simulink model "example_CondensingBoiler"  (R2016b)
settings: Solver=ode45  StartTime=0.0  StopTime=1*24*3600  MaxStep=600  RelTol=1e-4  AbsTol=1e-5  EnableMultiTasking=on
libraries: carnot x6, simulink x2
settings Model: Creator=drhf  LastModifiedBy=drhf
settings DataIOCC: LimitDataPoints=on  SaveFormat=Array
settings OptimizationCC: DefaultParameterBehavior=Inlined  ExpressionDepthLimit=2147483647  LifeSpan=inf
settings DebuggingCC: SolverPrmCheckMsg=warning  UniqueDataStoreMsg=error  StateNameClashWarn=warning  SFUnexpectedBacktrackingDiag=warning  SFNoUnconditionalDefaultTransitionDiag=warning  SFExecutionAtInitializationDiag=none
settings HardwareCC: ProdBitPerPointer=32  ProdBitPerSizeT=32  ProdBitPerPtrDiffT=32  ProdLargestAtomicFloat=None  ProdIntDivRoundTo=Undefined  ProdEndianess=Unspecified  ProdWordSize=32  ProdHWDeviceType=32-bit Generic
settings ModelReferenceCC: PropagateSignalLabelsOutOfModel=off
settings GRTTargetCC: TargetLangStandard=C89/C90 (ANSI)  GeneratePreprocessorConditionals=Disable all  CombineOutputUpdateFcns=off  GRTInterface=on
settings ConfigComp: CovMetricSettings=dw  CovHtmlReporting=on  CovSaveCumulativeToWorkspaceVar=on  CovSaveSingleToWorkspaceVar=on  CovExternalEMLEnable=off

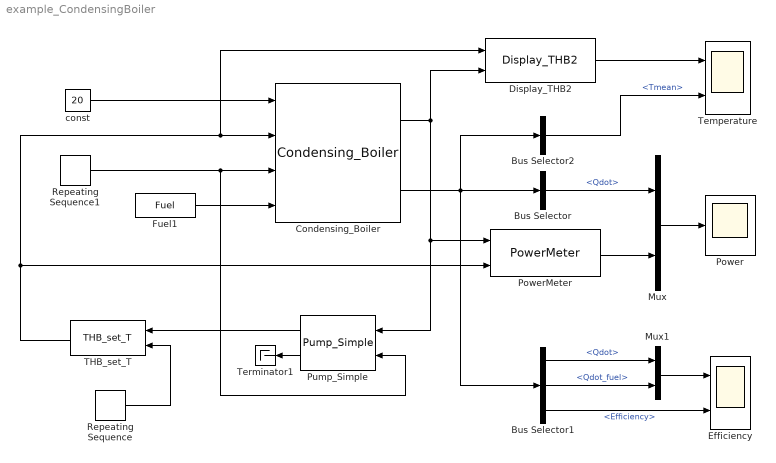
== system example_CondensingBoiler ==
  Bus Selector : BusSelector  OutputSignals=Qdot
  Bus Selector1 : BusSelector  OutputSignals=Qdot,eco.Qdot_fuel,eco.Efficiency
  Bus Selector2 : BusSelector  OutputSignals=Tmean
  Condensing_Boiler : carnot/Source/Boiler/Condensing_Boiler  Pgas=20e3  U=3  vol=0.02  electricPower=[20 120]  relativeQdot=[0.25 1]  whichTforEfficiency=mean of inlet and outlet temperature  temperatures="[40  70]"  efficiency=[1.05 0.95; 1.0 0.9]  lin=10  qua=100  Tini=20  nodes=1
  Display_THB2 : carnot/Outputs/Display_THB2  t=on  m=off  p=off  id=off  mix=off  d=off
  Efficiency : Scope  NumInputPorts=2
  Fuel1 : carnot/Source/Energy/Fuel  ft=1  t=20  ls=1  p=1e5  h_values=[5.14e7 5.69e7]  tc=45  price=1  mass=[0.33 0.67 0 0 0 0]
  Mux : Mux  Inputs=2
  Mux1 : Mux  Inputs=2
  Power : Scope
  PowerMeter : carnot/Control/PowerMeter
  Pump_Simple : carnot/Hydraulics/Pump_Simple  mdotmax=1600/3600  dia=0.0157  power=30  fluid_id=Water  mix=0  p0=3e5
  Repeating Sequence : simulink/Sources/Repeating Sequence  rep_seq_t=[0 12 24]*3600  rep_seq_y=[30 70 30]
  Repeating Sequence1 : simulink/Sources/Repeating Sequence  rep_seq_t=[0 6 12]*3600  rep_seq_y=[1 1 1] %[0.25 1 0.25]
  THB_set_T : carnot/Source/Simple/THB_set_T
  Temperature : Scope  NumInputPorts=2
  Terminator1 : Terminator
  const : Constant  Value=20
  wires:
  const/1 -> Condensing_Boiler/1
  THB_set_T/1 -> Condensing_Boiler/2, Display_THB2/1, PowerMeter/2
  Repeating Sequence1/1 -> Condensing_Boiler/3, Pump_Simple/2
  Fuel1/1 -> Condensing_Boiler/4
  Condensing_Boiler/1 -> Pump_Simple/1, PowerMeter/1, Display_THB2/2
  Display_THB2/1 -> Temperature/1
  Condensing_Boiler/2 -> Bus Selector/1, Bus Selector1/1, Bus Selector2/1
  Mux/1 -> Power/1
  PowerMeter/1 -> Mux/2
  Bus Selector/1 -> Mux/1  "<Qdot>"
  Pump_Simple/1 -> THB_set_T/1
  Pump_Simple/2 -> Terminator1/1
  Repeating Sequence/1 -> THB_set_T/2
  Bus Selector1/2 -> Mux1/2  "<Qdot_fuel>"
  Bus Selector1/1 -> Mux1/1  "<Qdot>"
  Mux1/1 -> Efficiency/1
  Bus Selector1/3 -> Efficiency/2  "<Efficiency>"
  Bus Selector2/1 -> Temperature/2  "<Tmean>"
